simulink model "PV2"  (R2014a)
settings: Solver=ode45  StartTime=0.0  StopTime=10.0  RelTol=1e-3
undefined symbols (not defined in the file): Io, K_IA, Rs, Rsh, sigbuilder_block, T
settings Model: Creator=HP  LastModifiedBy=HP

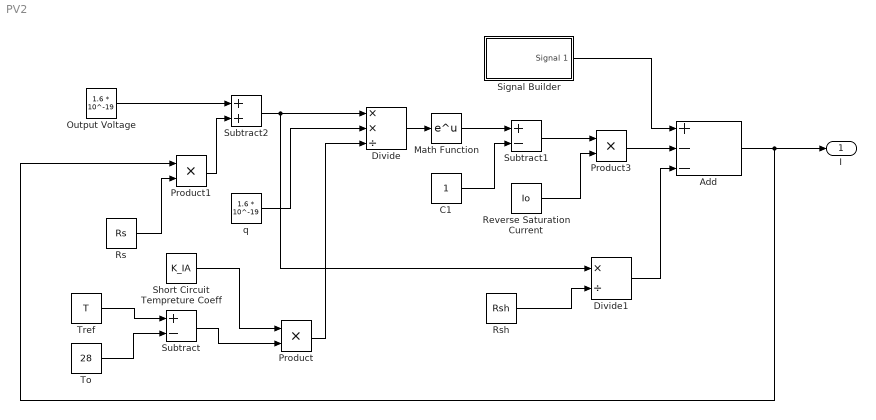
== system PV2 ==
  Add : Sum  Inputs=+--
  "C1 " : Constant
  Divide : Product  Inputs=**/
  Divide1 : Product  Inputs=*/
  Math Function : Math  SaturateOnIntegerOverflow=on
  Output Voltage : Constant  Value=1.6 * 10^-19
  Product : Product
  Product1 : Product
  Product3 : Product
  Reverse Saturation Current : Constant  Value=Io
  "Rs " : Constant  Value=Rs
  Rsh : Constant  Value=Rsh
  "Short Circuit Tempreture Coeff " : Constant  Value=K_IA
  Signal Builder : Subsystem  Tag=STV Subsys  LoadFcn=sigbuilder_block('load');  StartFcn=sigbuilder_block('start');  StopFcn=sigbuilder_block('stop');  ClipboardFcn=sigbuilder_block('clipboard');  mask(Sigbuilder block){}
      mask help: Simulink:masks:SigbuilderBlock_MD
      mask init:
      | if ~strcmp(get_param(bdroot(gcbh),'SimulationStatus'),'stopped') tuvar = sigbuilder_block('maskInit'); end
      settings: CopyFcn=sigbuilder_block('copy');  DeleteFcn=sigbuilder_block('delete');  ModelCloseFcn=sigbuilder_block('modelClose');  PreSaveFcn=sigbuilder_block('preSave');  PauseFcn=sigbuilder_block('pause');  ContinueFcn=sigbuilder_block('continue');  NameChangeFcn=sigbuilder_block('namechange');  OpenFcn=sigbuilder_block('open',[437.25 118.5 550.5 394.5 ]);  CloseFcn=sigbuilder_block('close');
      mask Display: plot(0, 0, 100, 100,[2, 2, 32, 32, 2], [68, 8, 8, 68, 68],[32, 2], [38, 38], [32, 19, 2],[53, 60, 44], [32, 17, 17, 2],[16, 16, 31, 31]);txt = getActiveGroup(gcbh);text(2, 100, txt,'verticalAlignment', 'top');
  Subtract : Sum  Inputs=+-
  Subtract1 : Sum  Inputs=+-
  Subtract2 : Sum
  To : Constant  Value=28
  "Tref " : Constant  Value=T
  q : Constant  Value=1.6 * 10^-19
  I : Outport
  wires:
  "Tref "/1 -> Subtract/1
  To/1 -> Subtract/2
  "Short Circuit Tempreture Coeff "/1 -> Product/1
  Subtract/1 -> Product/2
  Product/1 -> Divide/3
  Signal Builder/1(Signal 1) -> Add/1
  Divide/1 -> Math Function/1
  Math Function/1 -> Subtract1/1
  "C1 "/1 -> Subtract1/2
  Product3/1 -> Add/2
  Subtract1/1 -> Product3/1
  Reverse Saturation Current/1 -> Product3/2
  Product1/1 -> Subtract2/2
  Add/1 -> Product1/1, I/1
  "Rs "/1 -> Product1/2
  Subtract2/1 -> Divide1/1, Divide/1
  q/1 -> Divide/2
  Rsh/1 -> Divide1/2
  Divide1/1 -> Add/3
  Output Voltage/1 -> Subtract2/1

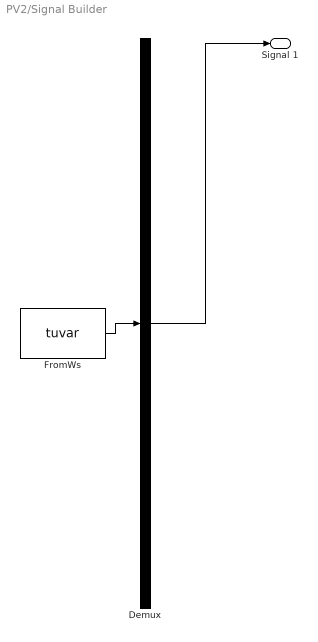
== system PV2/Signal Builder ==
  Demux : Demux  Tag=STV Demux  Outputs=1
  FromWs : FromWorkspace  Tag=STV FromWs  VariableName=tuvar  SampleTime=0
      SigBuilderData=|
      | common.afterFinalStr = 'Extrapolate'
      | common.sampleTime = 0
      | dataSet.timeRange = [0 10]
      | dataSet.name = 'Group 1'
      | sbobj.Groups.Name = 'Group 1'
      | sbobj.Groups.Signals.Name = 'Signal 1'
      | sbobj.Groups.Signals.XData = [0 4 4 6 6 10]
      | sbobj.Groups.Signals.YData = [2.99 2.99 2.64 2.64 1.9 1.9]
  Signal 1 : Outport  Tag=STV Outport
  wires:
  Demux/1 -> Signal 1/1
  FromWs/1 -> Demux/1
